simulink model "ParkingMeterSystem"  (R2023a)
settings: Solver=FixedStepDiscrete  StartTime=0.0  StopTime=Inf  FixedStep=SAMPLING_TIME  RelTol=1e-3
PreLoadFcn:
  | % Open the external C# interface
  | startGUI();
PostLoadFcn:
  | warning('off','Simulink:SimulationPacing:UnsupportedSimulationMode');
InitFcn:
  | % Assign the right data dictionary based on the selected mode to run
  | assignDataDictionary;
StartFcn:
  | disp('Referenced models loaded');
undefined symbols (not defined in the file): D1, P
CloseFcn:
  | % Close the external C# interface
  | closeGUI();
settings Model: DataDictionary=Parameters.sldd  Creator=sebas  LastModifiedBy=sdupertu
settings DataIOCC: ReturnWorkspaceOutputs=off
settings OptimizationCC: DefaultParameterBehavior=Inlined  EnhancedBackFolding=on  PassReuseOutputArgsAs=Individual arguments  ZeroExternalMemoryAtStartup=off  ZeroInternalMemoryAtStartup=off  OptimizeBlockOrder=speed  DifferentSizesBufferReuse=on  OptimizationCustomize=off  EfficientTunableParamExpr=on
settings DebuggingCC: ParameterTunabilityLossMsg=error
settings SFSimCC: MATLABDynamicMemAlloc=off
settings RTWCC: Description=Embedded Coder  SystemTargetFile=ert.tlc  TemplateMakefile=ert_default_tmf
settings CodeAppCC: ForceParamTrailComments=on  IgnoreCustomStorageClasses=off  MaxIdLength=61  OperatorAnnotations=on  SimulinkDataObjDesc=on  SFDataObjDesc=on  InsertBlockDesc=on
settings ERTTargetCC: TargetLangStandard=C99 (ISO)  GenerateSampleERTMain=on  IncludeMdlTerminateFcn=off  RemoveDisableFunc=on  InlinedParameterPlacement=NonHierarchical  ERTCustomFileTemplate=example_file_process.tlc

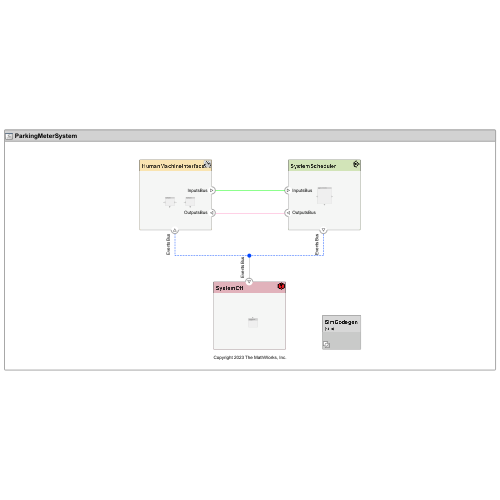
[thumbnail: Simulink's stored preview of the top-level diagram]
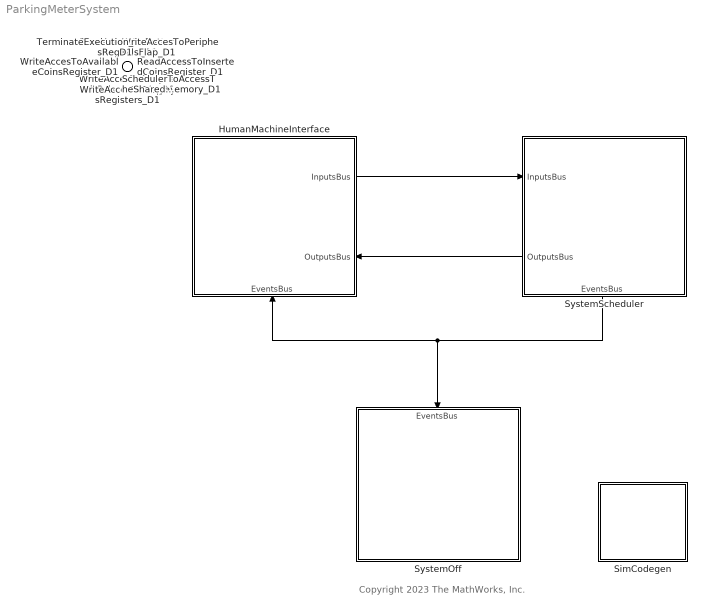
== system ParkingMeterSystem ==
  note: Copyright 2023 The MathWorks, Inc.
  WriteAccesToPeripheralsPulseGeneration_D1 : Inport  OutputFunctionCall=on
  ReadAccessToButtonsRegister_D1 : Inport  Port=2  OutputFunctionCall=on
  ReadAccessToInsertedCoinsRegister_D1 : Inport  Port=3  OutputFunctionCall=on
  WriteAccesToAvailableCoinsRegister_D1 : Inport  Port=4  OutputFunctionCall=on
  WriteAccesToDisplaysRegisters_D1 : Inport  Port=5  OutputFunctionCall=on
  WriteAccesToPeripheralsFlap_D1 : Inport  Port=6  OutputFunctionCall=on
  TerminateExecution_D1 : Inport  Port=7  OutputFunctionCall=on
  SchedulerToAccessTheSharedMemory_D1 : Inport  Port=8  OutputFunctionCall=on
  HumanMachineInterface : Subsystem
      settings: PortSchema="{\"entries\":[{\"content\":{\"headerSize\":26,\"margin\":15,\"minimumSpacing\":25,\"sides\":[{\"content\":{},\"type\":\"ConnectorPlacement.EquallySpacedRectSide\",\"uuid\":\"be809503-f1ea-4380-8942-33d79f2ad371\"},{\"content\":{\"connectorIds\":[\"Out1\",\"In2\"],\"side\":\"RIGHT\"},\"type\":\"ConnectorPlacement.EquallySpacedRectSide\",\"uuid\":\"d20c5475-d043-4994-ac49-3eb74728e760\"},{\"content\":{\"side\":\"TOP\"},\"type\":\"ConnectorPlacement.EquallySpacedRectSide\",\"uuid\":\"367a4a40-2fef-41b1-a218-3cfa4d79ed8f\"},{\"content\":{\"connectorIds\":[\"In1\"],\"side\":\"BOTTOM\"},\"type\":\"ConnectorPlacement.EquallySpacedRectSide\",\"uuid\":\"ad45a532-4028-4d32-9ed1-5493ed102a58\"}]},\"type\":\"ConnectorPlacement.EquallySpacedConnector\",\"uuid\":\"eb419f36-354b-4c4e-9a9c-8f8f96d7f82d\"}],\"packageUris\":[\"http://schema.mathworks.com/mf0/Connector/R2020b\"],\"version\":\"1.0\"}"
  SimCodegen : Subsystem  Variant=on  VariantControlMode=sim codegen switching
      settings: PortSchema="{\"entries\":[{\"content\":{\"headerSize\":38,\"margin\":15,\"minimumSpacing\":25,\"sides\":[{\"content\":{},\"type\":\"ConnectorPlacement.EquallySpacedRectSide\",\"uuid\":\"484e6def-1bba-4c5a-88bb-22e3a3a080bf\"},{\"content\":{\"side\":\"RIGHT\"},\"type\":\"ConnectorPlacement.EquallySpacedRectSide\",\"uuid\":\"1abd4651-a862-4957-abe2-c424248ffbbe\"},{\"content\":{\"side\":\"TOP\"},\"type\":\"ConnectorPlacement.EquallySpacedRectSide\",\"uuid\":\"2cb6a0bd-4256-480f-af1c-99a1cd270137\"}]},\"type\":\"ConnectorPlacement.EquallySpacedConnector\",\"uuid\":\"f5333b10-f4cf-45ce-ba25-bfe8cb6f3bde\"}],\"packageUris\":[\"http://schema.mathworks.com/mf0/Connector/R2020b\"],\"version\":\"1.0\"}"
  SystemOff : Subsystem
      settings: PortSchema="{\"entries\":[{\"content\":{\"headerSize\":26,\"margin\":15,\"minimumSpacing\":25,\"sides\":[{\"content\":{},\"type\":\"ConnectorPlacement.EquallySpacedRectSide\",\"uuid\":\"2123d831-2173-4642-8d7d-b6b2d490bb10\"},{\"content\":{\"side\":\"RIGHT\"},\"type\":\"ConnectorPlacement.EquallySpacedRectSide\",\"uuid\":\"70a1346a-6760-45e5-891a-b0f2399f5c2b\"},{\"content\":{\"connectorIds\":[\"In1\"],\"side\":\"TOP\"},\"type\":\"ConnectorPlacement.EquallySpacedRectSide\",\"uuid\":\"2af5cf57-aa76-4481-bc76-70542c0aed16\"}]},\"type\":\"ConnectorPlacement.EquallySpacedConnector\",\"uuid\":\"23925f50-19d1-46ca-b951-25f232ffb553\"}],\"packageUris\":[\"http://schema.mathworks.com/mf0/Connector/R2020b\"],\"version\":\"1.0\"}"
  SystemScheduler : Subsystem
      settings: PortSchema="{\"entries\":[{\"content\":{\"headerSize\":26,\"margin\":15,\"minimumSpacing\":25,\"sides\":[{\"content\":{\"connectorIds\":[\"In1\",\"Out2\"]},\"type\":\"ConnectorPlacement.EquallySpacedRectSide\",\"uuid\":\"be809503-f1ea-4380-8942-33d79f2ad371\"},{\"content\":{\"side\":\"RIGHT\"},\"type\":\"ConnectorPlacement.EquallySpacedRectSide\",\"uuid\":\"d20c5475-d043-4994-ac49-3eb74728e760\"},{\"content\":{\"side\":\"TOP\"},\"type\":\"ConnectorPlacement.EquallySpacedRectSide\",\"uuid\":\"367a4a40-2fef-41b1-a218-3cfa4d79ed8f\"},{\"content\":{\"connectorIds\":[\"Out1\"],\"side\":\"BOTTOM\"},\"type\":\"ConnectorPlacement.EquallySpacedRectSide\",\"uuid\":\"599a3aa0-021a-4e17-bee6-5fef34730978\"}]},\"type\":\"ConnectorPlacement.EquallySpacedConnector\",\"uuid\":\"eb419f36-354b-4c4e-9a9c-8f8f96d7f82d\"}],\"packageUris\":[\"http://schema.mathworks.com/mf0/Connector/R2020b\"],\"version\":\"1.0\"}"
  wires:
  SystemScheduler/2(OutputsBus) -> HumanMachineInterface/2(OutputsBus)
  HumanMachineInterface/1(InputsBus) -> SystemScheduler/1(InputsBus)
  SystemScheduler/1(EventsBus) -> SystemOff/1(EventsBus), HumanMachineInterface/1(EventsBus)

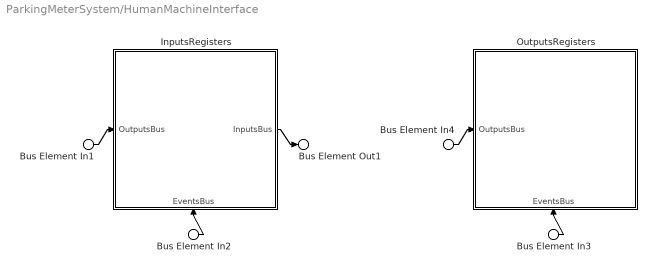
== system ParkingMeterSystem/HumanMachineInterface ==
  Bus Element In2 : Inport  PortName=EventsBus
  Bus Element In3 : Inport  PortName=EventsBus
  Bus Element In1 : Inport  Port=2  PortName=OutputsBus
  Bus Element In4 : Inport  Port=2  PortName=OutputsBus
  InputsRegisters : Subsystem
      settings: PortSchema="{\"entries\":[{\"content\":{\"headerSize\":26,\"margin\":15,\"minimumSpacing\":25,\"sides\":[{\"content\":{\"connectorIds\":[\"In2\"]},\"type\":\"ConnectorPlacement.EquallySpacedRectSide\",\"uuid\":\"be809503-f1ea-4380-8942-33d79f2ad371\"},{\"content\":{\"connectorIds\":[\"Out1\"],\"side\":\"RIGHT\"},\"type\":\"ConnectorPlacement.EquallySpacedRectSide\",\"uuid\":\"d20c5475-d043-4994-ac49-3eb74728e760\"},{\"content\":{\"side\":\"TOP\"},\"type\":\"ConnectorPlacement.EquallySpacedRectSide\",\"uuid\":\"367a4a40-2fef-41b1-a218-3cfa4d79ed8f\"},{\"content\":{\"connectorIds\":[\"In1\"],\"side\":\"BOTTOM\"},\"type\":\"ConnectorPlacement.EquallySpacedRectSide\",\"uuid\":\"42433694-7d38-411e-8c36-0d107f91df78\"}]},\"type\":\"ConnectorPlacement.EquallySpacedConnector\",\"uuid\":\"eb419f36-354b-4c4e-9a9c-8f8f96d7f82d\"}],\"packageUris\":[\"http://schema.mathworks.com/mf0/Connector/R2020b\"],\"version\":\"1.0\"}"
  OutputsRegisters : Subsystem
      settings: PortSchema="{\"entries\":[{\"content\":{\"headerSize\":26,\"margin\":15,\"minimumSpacing\":25,\"sides\":[{\"content\":{\"connectorIds\":[\"In1\"]},\"type\":\"ConnectorPlacement.EquallySpacedRectSide\",\"uuid\":\"be809503-f1ea-4380-8942-33d79f2ad371\"},{\"content\":{\"side\":\"RIGHT\"},\"type\":\"ConnectorPlacement.EquallySpacedRectSide\",\"uuid\":\"d20c5475-d043-4994-ac49-3eb74728e760\"},{\"content\":{\"side\":\"TOP\"},\"type\":\"ConnectorPlacement.EquallySpacedRectSide\",\"uuid\":\"367a4a40-2fef-41b1-a218-3cfa4d79ed8f\"},{\"content\":{\"connectorIds\":[\"In2\"],\"side\":\"BOTTOM\"},\"type\":\"ConnectorPlacement.EquallySpacedRectSide\",\"uuid\":\"9411f4e0-b09e-492c-9d7b-7970a952076c\"}]},\"type\":\"ConnectorPlacement.EquallySpacedConnector\",\"uuid\":\"eb419f36-354b-4c4e-9a9c-8f8f96d7f82d\"}],\"packageUris\":[\"http://schema.mathworks.com/mf0/Connector/R2020b\"],\"version\":\"1.0\"}"
  Bus Element Out1 : Outport  PortName=InputsBus
  wires:
  Bus Element In1/1 -> InputsRegisters/2(OutputsBus)
  InputsRegisters/1(InputsBus) -> Bus Element Out1/1
  Bus Element In2/1 -> InputsRegisters/1(EventsBus)
  Bus Element In3/1 -> OutputsRegisters/2(EventsBus)
  Bus Element In4/1 -> OutputsRegisters/1(OutputsBus)

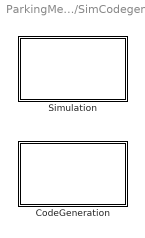
== system ParkingMeterSystem/SimCodegen ==
  CodeGeneration : Subsystem  VariantControl=(codegen)
      settings: PortSchema="{\"entries\":[{\"content\":{\"headerSize\":26,\"margin\":15,\"minimumSpacing\":25,\"sides\":[{\"content\":{},\"type\":\"ConnectorPlacement.EquallySpacedRectSide\",\"uuid\":\"4d0f3abe-5f09-4a53-b406-96a471b1431e\"},{\"content\":{\"side\":\"RIGHT\"},\"type\":\"ConnectorPlacement.EquallySpacedRectSide\",\"uuid\":\"0cf42196-2b1b-4979-9cbd-e482e09063e4\"},{\"content\":{\"side\":\"TOP\"},\"type\":\"ConnectorPlacement.EquallySpacedRectSide\",\"uuid\":\"a0d8888a-19a5-4fde-bda5-702eb867e877\"}]},\"type\":\"ConnectorPlacement.EquallySpacedConnector\",\"uuid\":\"80091a88-1c7a-41b6-b9b6-db6eef13398c\"}],\"packageUris\":[\"http://schema.mathworks.com/mf0/Connector/R2020b\"],\"version\":\"1.0\"}"
  Simulation : Subsystem  VariantControl=(sim)
      settings: PortSchema="{\"entries\":[{\"content\":{\"headerSize\":26,\"margin\":15,\"minimumSpacing\":25,\"sides\":[{\"content\":{},\"type\":\"ConnectorPlacement.EquallySpacedRectSide\",\"uuid\":\"4d0f3abe-5f09-4a53-b406-96a471b1431e\"},{\"content\":{\"side\":\"RIGHT\"},\"type\":\"ConnectorPlacement.EquallySpacedRectSide\",\"uuid\":\"0cf42196-2b1b-4979-9cbd-e482e09063e4\"},{\"content\":{\"side\":\"TOP\"},\"type\":\"ConnectorPlacement.EquallySpacedRectSide\",\"uuid\":\"a0d8888a-19a5-4fde-bda5-702eb867e877\"}]},\"type\":\"ConnectorPlacement.EquallySpacedConnector\",\"uuid\":\"80091a88-1c7a-41b6-b9b6-db6eef13398c\"}],\"packageUris\":[\"http://schema.mathworks.com/mf0/Connector/R2020b\"],\"version\":\"1.0\"}"

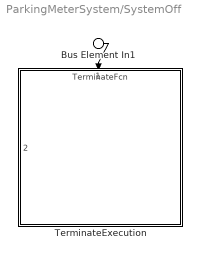
== system ParkingMeterSystem/SystemOff ==
  Bus Element In1 : Inport  PortName=EventsBus
  TerminateExecution : ModelReference  ModelNameDialog=TerminateFcn  SimulationMode=Normal  ScheduleRates=on  CachedPortDiscreteRates=[0.001]  ModelEventPortInfo=P:D1[0.001][0][0]  ModelReferenceVersion=8.13
      settings: PortSchema="{\"entries\":[{\"content\":{\"headerSize\":38,\"margin\":15,\"minimumSpacing\":25,\"sides\":[{\"content\":{},\"type\":\"ConnectorPlacement.EquallySpacedRectSide\",\"uuid\":\"be809503-f1ea-4380-8942-33d79f2ad371\"},{\"content\":{\"side\":\"RIGHT\"},\"type\":\"ConnectorPlacement.EquallySpacedRectSide\",\"uuid\":\"d20c5475-d043-4994-ac49-3eb74728e760\"},{\"content\":{\"connectorIds\":[\"In1\"],\"side\":\"TOP\"},\"type\":\"ConnectorPlacement.EquallySpacedRectSide\",\"uuid\":\"367a4a40-2fef-41b1-a218-3cfa4d79ed8f\"},{\"content\":{\"connectorIds\":[\"In2\"],\"side\":\"HIDDEN\"},\"type\":\"ConnectorPlacement.EquallySpacedRectSide\",\"uuid\":\"2b7aa608-e8c7-4427-8225-0280e4f358e9\"}]},\"type\":\"ConnectorPlacement.EquallySpacedConnector\",\"uuid\":\"eb419f36-354b-4c4e-9a9c-8f8f96d7f82d\"}],\"packageUris\":[\"http://schema.mathworks.com/mf0/Connector/R2020b\"],\"version\":\"1.0\"}"
  wires:
  Bus Element In1/1 -> TerminateExecution/1

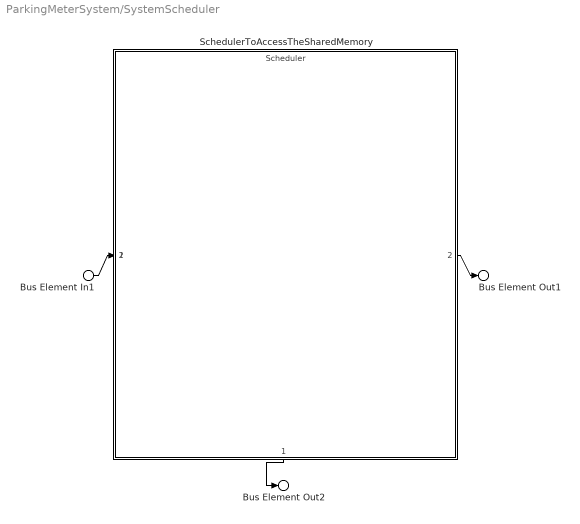
== system ParkingMeterSystem/SystemScheduler ==
  Bus Element In1 : Inport  PortName=InputsBus
  SchedulerToAccessTheSharedMemory : ModelReference  ModelNameDialog=Scheduler  SimulationMode=Normal  ScheduleRates=on  CachedPortDiscreteRates=[0.001]  ModelEventPortInfo=P:D1[0.001][0][0]  ModelReferenceVersion=8.20
      settings: PortSchema="{\"entries\":[{\"content\":{\"headerSize\":38,\"margin\":15,\"minimumSpacing\":25,\"sides\":[{\"content\":{\"connectorIds\":[\"In1\"]},\"type\":\"ConnectorPlacement.EquallySpacedRectSide\",\"uuid\":\"be809503-f1ea-4380-8942-33d79f2ad371\"},{\"content\":{\"connectorIds\":[\"Out2\"],\"side\":\"RIGHT\"},\"type\":\"ConnectorPlacement.EquallySpacedRectSide\",\"uuid\":\"d20c5475-d043-4994-ac49-3eb74728e760\"},{\"content\":{\"side\":\"TOP\"},\"type\":\"ConnectorPlacement.EquallySpacedRectSide\",\"uuid\":\"367a4a40-2fef-41b1-a218-3cfa4d79ed8f\"},{\"content\":{\"connectorIds\":[\"Out1\"],\"side\":\"BOTTOM\"},\"type\":\"ConnectorPlacement.EquallySpacedRectSide\",\"uuid\":\"fb86e00b-f9c7-4f3f-8cbd-dd4de8ac92df\"},{\"content\":{\"connectorIds\":[\"In2\"],\"side\":\"HIDDEN\"},\"type\":\"ConnectorPlacement.EquallySpacedRectSide\",\"uuid\":\"74e265bb-5a4f-4039-8bd9-f78af680f503\"}]},\"type\":\"ConnectorPlacement.EquallySpacedConnector\",\"uuid\":\"eb419f36-354b-4c4e-9a9c-8f8f96d7f82d\"}],\"packageUris\":[\"http://schema.mathworks.com/mf0/Connector/R2020b\"],\"version\":\"1.0\"}"
  Bus Element Out2 : Outport  PortName=EventsBus
  Bus Element Out1 : Outport  Port=2  PortName=OutputsBus
  wires:
  Bus Element In1/1 -> SchedulerToAccessTheSharedMemory/1
  SchedulerToAccessTheSharedMemory/1 -> Bus Element Out2/1
  SchedulerToAccessTheSharedMemory/2 -> Bus Element Out1/1

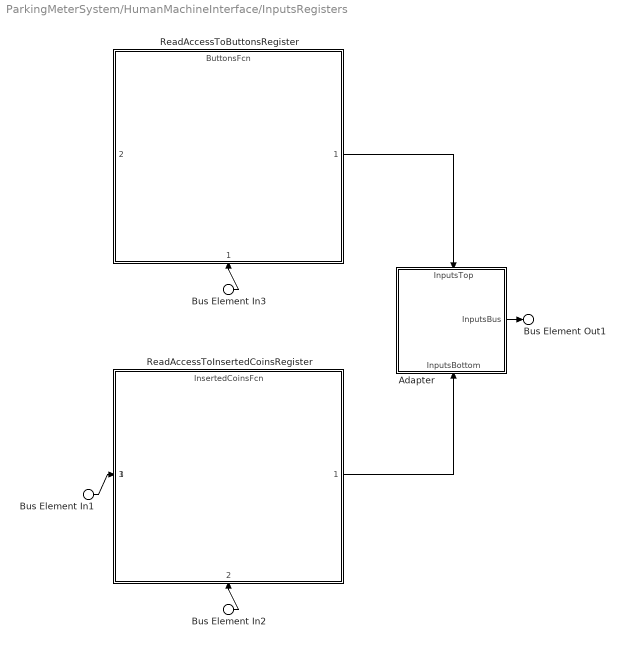
== system ParkingMeterSystem/HumanMachineInterface/InputsRegisters ==
  Bus Element In2 : Inport  PortName=EventsBus
  Bus Element In3 : Inport  PortName=EventsBus
  Bus Element In1 : Inport  Port=2  PortName=OutputsBus
  Adapter : Subsystem
      settings: PortSchema="{\"entries\":[{\"content\":{\"margin\":10,\"minimumSpacing\":15,\"sides\":[{\"content\":{},\"type\":\"ConnectorPlacement.EquallySpacedRectSide\",\"uuid\":\"2123d831-2173-4642-8d7d-b6b2d490bb10\"},{\"content\":{\"connectorIds\":[\"Out1\"],\"side\":\"RIGHT\"},\"type\":\"ConnectorPlacement.EquallySpacedRectSide\",\"uuid\":\"70a1346a-6760-45e5-891a-b0f2399f5c2b\"},{\"content\":{\"connectorIds\":[\"In1\"],\"side\":\"TOP\"},\"type\":\"ConnectorPlacement.EquallySpacedRectSide\",\"uuid\":\"2af5cf57-aa76-4481-bc76-70542c0aed16\"},{\"content\":{\"connectorIds\":[\"In2\"],\"side\":\"BOTTOM\"},\"type\":\"ConnectorPlacement.EquallySpacedRectSide\",\"uuid\":\"ba64882b-3141-4ded-b49d-bd7c6c693442\"}]},\"type\":\"ConnectorPlacement.EquallySpacedConnector\",\"uuid\":\"23925f50-19d1-46ca-b951-25f232ffb553\"}],\"packageUris\":[\"http://schema.mathworks.com/mf0/Connector/R2020b\"],\"version\":\"1.0\"}"
  ReadAccessToButtonsRegister : ModelReference  ModelNameDialog=ButtonsFcn  SimulationMode=Normal  ScheduleRates=on  CachedPortDiscreteRates=[0.001]  ModelEventPortInfo=P:D1[0.001][0][0]  ModelReferenceVersion=8.11
      settings: PortSchema="{\"entries\":[{\"content\":{\"headerSize\":38,\"margin\":15,\"minimumSpacing\":25,\"sides\":[{\"content\":{},\"type\":\"ConnectorPlacement.EquallySpacedRectSide\",\"uuid\":\"be809503-f1ea-4380-8942-33d79f2ad371\"},{\"content\":{\"connectorIds\":[\"Out1\"],\"side\":\"RIGHT\"},\"type\":\"ConnectorPlacement.EquallySpacedRectSide\",\"uuid\":\"d20c5475-d043-4994-ac49-3eb74728e760\"},{\"content\":{\"side\":\"TOP\"},\"type\":\"ConnectorPlacement.EquallySpacedRectSide\",\"uuid\":\"367a4a40-2fef-41b1-a218-3cfa4d79ed8f\"},{\"content\":{\"connectorIds\":[\"In1\"],\"side\":\"BOTTOM\"},\"type\":\"ConnectorPlacement.EquallySpacedRectSide\",\"uuid\":\"20a3fabb-dc20-4c8a-b758-ffeffe12cb5d\"},{\"content\":{\"connectorIds\":[\"In2\"],\"side\":\"HIDDEN\"},\"type\":\"ConnectorPlacement.EquallySpacedRectSide\",\"uuid\":\"619db0d7-0664-4085-915a-a74ff553ccfa\"}]},\"type\":\"ConnectorPlacement.EquallySpacedConnector\",\"uuid\":\"eb419f36-354b-4c4e-9a9c-8f8f96d7f82d\"}],\"packageUris\":[\"http://schema.mathworks.com/mf0/Connector/R2020b\"],\"version\":\"1.0\"}"
  ReadAccessToInsertedCoinsRegister : ModelReference  ModelNameDialog=InsertedCoinsFcn  SimulationMode=Normal  ScheduleRates=on  CachedPortDiscreteRates=[0.001]  ModelEventPortInfo=P:D1[0.001][0][0]  ModelReferenceVersion=8.13
      settings: PortSchema="{\"entries\":[{\"content\":{\"headerSize\":38,\"margin\":15,\"minimumSpacing\":25,\"sides\":[{\"content\":{\"connectorIds\":[\"In1\"]},\"type\":\"ConnectorPlacement.EquallySpacedRectSide\",\"uuid\":\"be809503-f1ea-4380-8942-33d79f2ad371\"},{\"content\":{\"connectorIds\":[\"Out1\"],\"side\":\"RIGHT\"},\"type\":\"ConnectorPlacement.EquallySpacedRectSide\",\"uuid\":\"d20c5475-d043-4994-ac49-3eb74728e760\"},{\"content\":{\"side\":\"TOP\"},\"type\":\"ConnectorPlacement.EquallySpacedRectSide\",\"uuid\":\"367a4a40-2fef-41b1-a218-3cfa4d79ed8f\"},{\"content\":{\"connectorIds\":[\"In2\"],\"side\":\"BOTTOM\"},\"type\":\"ConnectorPlacement.EquallySpacedRectSide\",\"uuid\":\"c4a18945-d859-4bf0-a176-342256d1a336\"},{\"content\":{\"connectorIds\":[\"In3\"],\"side\":\"HIDDEN\"},\"type\":\"ConnectorPlacement.EquallySpacedRectSide\",\"uuid\":\"52804af8-db2a-4760-b62b-c289e870e5aa\"}]},\"type\":\"ConnectorPlacement.EquallySpacedConnector\",\"uuid\":\"eb419f36-354b-4c4e-9a9c-8f8f96d7f82d\"}],\"packageUris\":[\"http://schema.mathworks.com/mf0/Connector/R2020b\"],\"version\":\"1.0\"}"
  Bus Element Out1 : Outport  PortName=InputsBus
  wires:
  Bus Element In1/1 -> ReadAccessToInsertedCoinsRegister/1
  Bus Element In2/1 -> ReadAccessToInsertedCoinsRegister/2
  Bus Element In3/1 -> ReadAccessToButtonsRegister/1
  Adapter/1(InputsBus) -> Bus Element Out1/1
  ReadAccessToButtonsRegister/1 -> Adapter/1(InputsTop)
  ReadAccessToInsertedCoinsRegister/1 -> Adapter/2(InputsBottom)

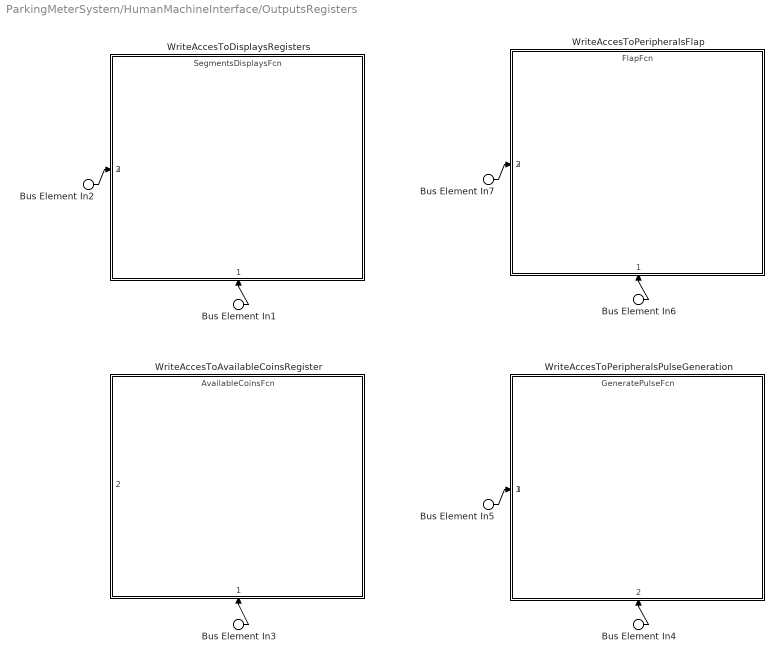
== system ParkingMeterSystem/HumanMachineInterface/OutputsRegisters ==
  Bus Element In2 : Inport  PortName=OutputsBus
  Bus Element In5 : Inport  PortName=OutputsBus
  Bus Element In7 : Inport  PortName=OutputsBus
  Bus Element In{1,3..4,6} (4 alike) : Inport  Port=2  PortName=EventsBus
  WriteAccesToAvailableCoinsRegister : ModelReference  ModelNameDialog=AvailableCoinsFcn  SimulationMode=Normal  ScheduleRates=on  CachedPortDiscreteRates=[0.001]  ModelEventPortInfo=P:D1[0.001][0][0]  ModelReferenceVersion=8.12
      settings: PortSchema="{\"entries\":[{\"content\":{\"headerSize\":38,\"margin\":15,\"minimumSpacing\":25,\"sides\":[{\"content\":{},\"type\":\"ConnectorPlacement.EquallySpacedRectSide\",\"uuid\":\"be809503-f1ea-4380-8942-33d79f2ad371\"},{\"content\":{\"side\":\"RIGHT\"},\"type\":\"ConnectorPlacement.EquallySpacedRectSide\",\"uuid\":\"d20c5475-d043-4994-ac49-3eb74728e760\"},{\"content\":{\"side\":\"TOP\"},\"type\":\"ConnectorPlacement.EquallySpacedRectSide\",\"uuid\":\"367a4a40-2fef-41b1-a218-3cfa4d79ed8f\"},{\"content\":{\"connectorIds\":[\"In1\"],\"side\":\"BOTTOM\"},\"type\":\"ConnectorPlacement.EquallySpacedRectSide\",\"uuid\":\"0ec21bd5-d732-4e1f-9584-045b5c892f8a\"},{\"content\":{\"connectorIds\":[\"In2\"],\"side\":\"HIDDEN\"},\"type\":\"ConnectorPlacement.EquallySpacedRectSide\",\"uuid\":\"3eb33428-824a-4da5-832a-2eacaca34f61\"}]},\"type\":\"ConnectorPlacement.EquallySpacedConnector\",\"uuid\":\"eb419f36-354b-4c4e-9a9c-8f8f96d7f82d\"}],\"packageUris\":[\"http://schema.mathworks.com/mf0/Connector/R2020b\"],\"version\":\"1.0\"}"
  WriteAccesToDisplaysRegisters : ModelReference  ModelNameDialog=SegmentsDisplaysFcn  SimulationMode=Normal  ScheduleRates=on  CachedPortDiscreteRates=[0.001]  ModelEventPortInfo=P:D1[0.001][0][0]  ModelReferenceVersion=8.12
      settings: PortSchema="{\"entries\":[{\"content\":{\"headerSize\":38,\"margin\":15,\"minimumSpacing\":25,\"sides\":[{\"content\":{\"connectorIds\":[\"In2\"]},\"type\":\"ConnectorPlacement.EquallySpacedRectSide\",\"uuid\":\"be809503-f1ea-4380-8942-33d79f2ad371\"},{\"content\":{\"side\":\"RIGHT\"},\"type\":\"ConnectorPlacement.EquallySpacedRectSide\",\"uuid\":\"d20c5475-d043-4994-ac49-3eb74728e760\"},{\"content\":{\"side\":\"TOP\"},\"type\":\"ConnectorPlacement.EquallySpacedRectSide\",\"uuid\":\"367a4a40-2fef-41b1-a218-3cfa4d79ed8f\"},{\"content\":{\"connectorIds\":[\"In1\"],\"side\":\"BOTTOM\"},\"type\":\"ConnectorPlacement.EquallySpacedRectSide\",\"uuid\":\"41896e6e-9ee0-46f4-85c5-427c3971bd92\"},{\"content\":{\"connectorIds\":[\"In3\"],\"side\":\"HIDDEN\"},\"type\":\"ConnectorPlacement.EquallySpacedRectSide\",\"uuid\":\"0339ac93-600c-466f-8072-11d736857049\"}]},\"type\":\"ConnectorPlacement.EquallySpacedConnector\",\"uuid\":\"eb419f36-354b-4c4e-9a9c-8f8f96d7f82d\"}],\"packageUris\":[\"http://schema.mathworks.com/mf0/Connector/R2020b\"],\"version\":\"1.0\"}"
  WriteAccesToPeripheralsFlap : ModelReference  ModelNameDialog=FlapFcn  SimulationMode=Normal  ScheduleRates=on  CachedPortDiscreteRates=[0.001]  ModelEventPortInfo=P:D1[0.001][0][0]  ModelReferenceVersion=8.12
      settings: PortSchema="{\"entries\":[{\"content\":{\"headerSize\":38,\"margin\":15,\"minimumSpacing\":25,\"sides\":[{\"content\":{\"connectorIds\":[\"In2\"]},\"type\":\"ConnectorPlacement.EquallySpacedRectSide\",\"uuid\":\"be809503-f1ea-4380-8942-33d79f2ad371\"},{\"content\":{\"side\":\"RIGHT\"},\"type\":\"ConnectorPlacement.EquallySpacedRectSide\",\"uuid\":\"d20c5475-d043-4994-ac49-3eb74728e760\"},{\"content\":{\"side\":\"TOP\"},\"type\":\"ConnectorPlacement.EquallySpacedRectSide\",\"uuid\":\"367a4a40-2fef-41b1-a218-3cfa4d79ed8f\"},{\"content\":{\"connectorIds\":[\"In1\"],\"side\":\"BOTTOM\"},\"type\":\"ConnectorPlacement.EquallySpacedRectSide\",\"uuid\":\"14e3096b-a6b9-4981-8345-e34eabc07420\"},{\"content\":{\"connectorIds\":[\"In3\"],\"side\":\"HIDDEN\"},\"type\":\"ConnectorPlacement.EquallySpacedRectSide\",\"uuid\":\"98d0f007-bbbb-419c-9a0b-eb95b9f54b7b\"}]},\"type\":\"ConnectorPlacement.EquallySpacedConnector\",\"uuid\":\"eb419f36-354b-4c4e-9a9c-8f8f96d7f82d\"}],\"packageUris\":[\"http://schema.mathworks.com/mf0/Connector/R2020b\"],\"version\":\"1.0\"}"
  WriteAccesToPeripheralsPulseGeneration : ModelReference  ModelNameDialog=GeneratePulseFcn  SimulationMode=Normal  ScheduleRates=on  CachedPortDiscreteRates=[0.15]  ModelEventPortInfo=P:D1[0.15][0][0]  ModelReferenceVersion=8.12
      settings: PortSchema="{\"entries\":[{\"content\":{\"headerSize\":38,\"margin\":15,\"minimumSpacing\":25,\"sides\":[{\"content\":{\"connectorIds\":[\"In1\"]},\"type\":\"ConnectorPlacement.EquallySpacedRectSide\",\"uuid\":\"be809503-f1ea-4380-8942-33d79f2ad371\"},{\"content\":{\"side\":\"RIGHT\"},\"type\":\"ConnectorPlacement.EquallySpacedRectSide\",\"uuid\":\"d20c5475-d043-4994-ac49-3eb74728e760\"},{\"content\":{\"side\":\"TOP\"},\"type\":\"ConnectorPlacement.EquallySpacedRectSide\",\"uuid\":\"367a4a40-2fef-41b1-a218-3cfa4d79ed8f\"},{\"content\":{\"connectorIds\":[\"In2\"],\"side\":\"BOTTOM\"},\"type\":\"ConnectorPlacement.EquallySpacedRectSide\",\"uuid\":\"a191c519-7795-4009-b1e2-432976e0f9f0\"},{\"content\":{\"connectorIds\":[\"In3\"],\"side\":\"HIDDEN\"},\"type\":\"ConnectorPlacement.EquallySpacedRectSide\",\"uuid\":\"c29be4a7-1c06-4825-ad5a-289e3e32d959\"}]},\"type\":\"ConnectorPlacement.EquallySpacedConnector\",\"uuid\":\"eb419f36-354b-4c4e-9a9c-8f8f96d7f82d\"}],\"packageUris\":[\"http://schema.mathworks.com/mf0/Connector/R2020b\"],\"version\":\"1.0\"}"
  wires:
  Bus Element In2/1 -> WriteAccesToDisplaysRegisters/2
  Bus Element In1/1 -> WriteAccesToDisplaysRegisters/1
  Bus Element In3/1 -> WriteAccesToAvailableCoinsRegister/1
  Bus Element In4/1 -> WriteAccesToPeripheralsPulseGeneration/2
  Bus Element In5/1 -> WriteAccesToPeripheralsPulseGeneration/1
  Bus Element In6/1 -> WriteAccesToPeripheralsFlap/1
  Bus Element In7/1 -> WriteAccesToPeripheralsFlap/2

== system ParkingMeterSystem/SimCodegen/CodeGeneration ==

== system ParkingMeterSystem/SimCodegen/Simulation ==

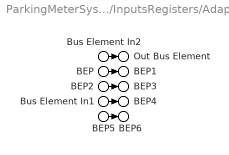
== system ParkingMeterSystem/HumanMachineInterface/InputsRegisters/Adapter ==
  Bus Element In2 : Inport  PortName=InputsTop  Element=green_pressed
  BEP : Inport  PortName=InputsTop  Element=red_pressed
  BEP2 : Inport  PortName=InputsTop  Element=master_switch
  Bus Element In1 : Inport  Port=2  PortName=InputsBottom  Element=coins_reg_value
  BEP5 : Inport  Port=2  PortName=InputsBottom  Element=temp_amount
  Out Bus Element : Outport  PortName=InputsBus  Element=green_pressed
  BEP1 : Outport  PortName=InputsBus  Element=red_pressed
  BEP3 : Outport  PortName=InputsBus  Element=master_switch
  BEP4 : Outport  PortName=InputsBus  Element=coins_reg_value
  BEP6 : Outport  PortName=InputsBus  Element=temp_amount
  wires:
  Bus Element In2/1 -> Out Bus Element/1
  BEP/1 -> BEP1/1
  BEP2/1 -> BEP3/1
  Bus Element In1/1 -> BEP4/1
  BEP5/1 -> BEP6/1
